simulink model "aerobalancin_modelo"  (R2025b)
settings: Solver=VariableStepAuto  StartTime=0.0  StopTime=40  FixedStep=1e-5  RelTol=1e-3
values from neighbouring files (symbols this model uses):
  d1 = 130.5e-3    (= 0.1305)    [Fuerzas.m]    (also in hinf.m)
  I = 1.3636e-4    (= 0.00013636)    [Fuerzas.m]    (also in hinf.m)
  k = (Wcp*d2-d1*Wm-e*Wb)    (= -0.00869250366)    [Fuerzas.m]    (also in hinf.m)
  Ka = m    (= 0.00012984)    [hinf.m]
  Kb = b    (= -0.0231)    [hinf.m]
  mu = 2e-04    (= 0.0002)    [Fuerzas.m]    (also in hinf.m = 0.0004)
  P_pwm_deg = series(Scale * P0, Act)    [hinf.m]
  T_ref = feedback(K*P_pwm_deg, 1)    [hinf.m]
undefined symbols (not defined in the file or in its folder): K
libraries: simulink_extras x3
settings Model: Creator=Gabriel Bojaca  LastModifiedBy=Gabriel Bojaca

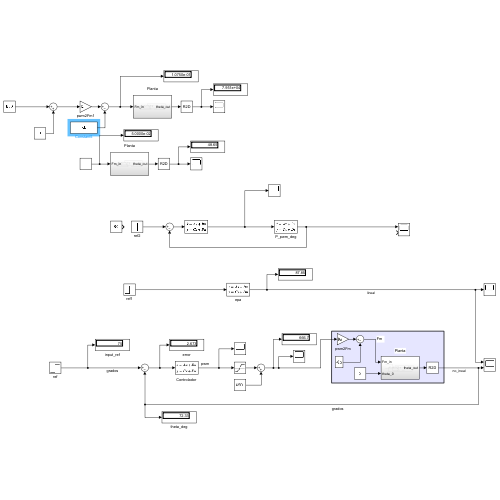
[thumbnail: Simulink's stored preview of the top-level diagram]
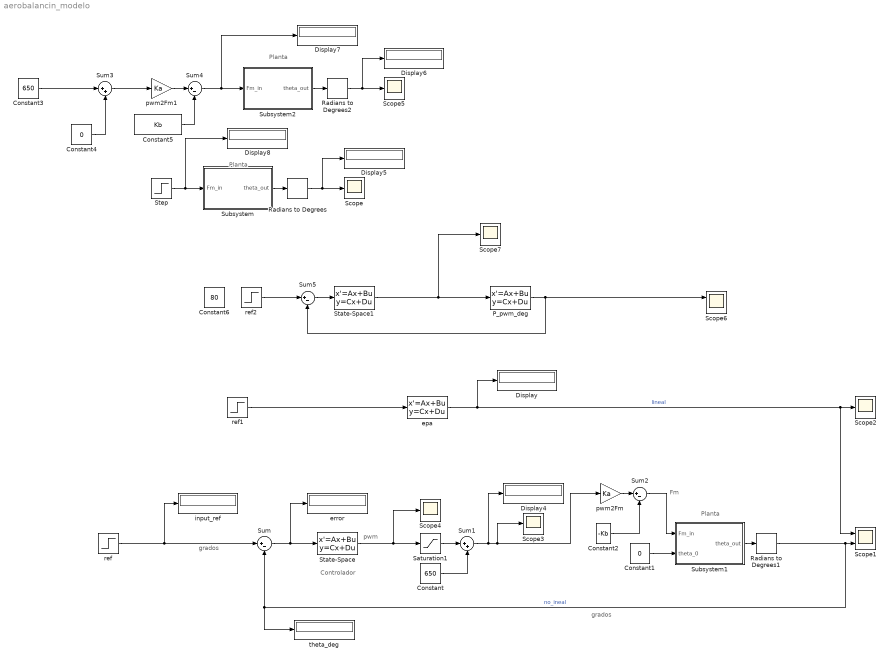
== system aerobalancin_modelo ==
  note: pwm
  note: Fm
  note: grados
  note: grados
  note: Planta
  note: Planta
  note: Controlador
  note: Planta
  Constant : Constant  Value=650
  Constant1 : Constant  Value=0
  Constant2 : Constant  Value=-Kb
  Constant3 : Constant  Value=650
  Constant4 : Constant  Value=0
  Constant5 : Constant  Value=Kb
  Constant6 : Constant  Value=80
  Display{,4..8} (6 alike) : Display
      Display7 settings: Format=short_e
      Display8 settings: Format=short_e
  P_pwm_deg : StateSpace  A=P_pwm_deg.A  B=P_pwm_deg.B  C=P_pwm_deg.C  D=P_pwm_deg.D  InitialCondition=0
  Radians to Degrees : simulink_extras/Transformations/Radians to Degrees
  Radians to Degrees1 : simulink_extras/Transformations/Radians to Degrees
  Radians to Degrees2 : simulink_extras/Transformations/Radians to Degrees
  Saturation1 : Saturate  UpperLimit=1023  LowerLimit=-1023  ZeroCross=off
  Scope{,2..5,7} (6 alike) : Scope
      Scope settings: ActiveDisplayYMinimum=-1  ActiveDisplayYMaximum=1
      Scope2 settings: ActiveDisplayYMinimum=79.481508887429072  ActiveDisplayYMaximum=97.233534907130334  DataLoggingVariableName=ScopeData2
      Scope3 settings: ActiveDisplayYMinimum=-1  ActiveDisplayYMaximum=1  DataLoggingVariableName=ScopeData3
      Scope4 settings: ActiveDisplayYMinimum=-86.058155781433356  ActiveDisplayYMaximum=157.82486783945171  DataLoggingVariableName=ScopeData4
      Scope5 settings: ActiveDisplayYMinimum=-227.29137035999565  ActiveDisplayYMaximum=925.661296141076  DataLoggingVariableName=ScopeData5
      Scope7 settings: ActiveDisplayYMinimum=-379.74870159092234  ActiveDisplayYMaximum=1124.590386355748  DataLoggingVariableName=ScopeData7
  Scope1 : Scope  NumInputPorts=2
      settings: ActiveDisplayYMinimum=-12.36574518282506  ActiveDisplayYMaximum=111.29170664542558
  Scope6 : Scope  NumInputPorts=2
      settings: ActiveDisplayYMinimum=-21.487013415649258  ActiveDisplayYMaximum=193.38312074084337  DataLoggingVariableName=ScopeData6
  State-Space : StateSpace  A=K.A  B=K.B  C=K.C  D=K.D  InitialCondition=0
  State-Space1 : StateSpace  A=K.A  B=K.B  C=K.C  D=K.D  InitialCondition=0
  Step : Step  After=50e-3  SampleTime=0
  Subsystem : Subsystem
  Subsystem1 : Subsystem
  Subsystem2 : Subsystem
  Sum{,2,4..5} (4 alike) : Sum  Inputs=|+-
  Sum1 : Sum  Inputs=|++
  Sum3 : Sum  Inputs=|++
  epa : StateSpace  A=T_ref.A  B=T_ref.B  C=T_ref.C  D=T_ref.D  InitialCondition=0
  error : Display
  input_ref : Display
  pwm2Fm : Gain  Gain=Ka
  pwm2Fm1 : Gain  Gain=Ka
  ref : Step  Time=20  Before=60  After=75  SampleTime=0
  ref1 : Step  Time=10  Before=77  After=85  SampleTime=0
  ref2 : Step  Time=0  Before=77  After=85  SampleTime=0
  theta_deg : Display
  wires:
  Subsystem/1(theta_out) -> Radians to Degrees/1
  Step/1 -> Display8/1, Subsystem/1(Fm_in)
  Subsystem1/1(theta_out) -> Radians to Degrees1/1
  Sum/1 -> State-Space/1, error/1
  Radians to Degrees1/1 -> Sum/2, theta_deg/1, Scope1/2  "no_ineal"
  ref/1 -> Sum/1, input_ref/1
  epa/1 -> Display/1, Scope1/1, Scope2/1  "lineal"
  State-Space/1 -> Saturation1/1, Scope4/1
  Sum1/1 -> Display4/1, pwm2Fm/1, Scope3/1
  Constant/1 -> Sum1/2
  Constant1/1 -> Subsystem1/2(theta_0)
  pwm2Fm/1 -> Sum2/1
  Sum2/1 -> Subsystem1/1(Fm_in)
  Constant2/1 -> Sum2/2
  Radians to Degrees/1 -> Display5/1, Scope/1
  Subsystem2/1(theta_out) -> Radians to Degrees2/1
  Radians to Degrees2/1 -> Display6/1, Scope5/1
  Sum4/1 -> Display7/1, Subsystem2/1(Fm_in)
  Sum3/1 -> pwm2Fm1/1
  Constant3/1 -> Sum3/1
  Constant4/1 -> Sum3/2
  pwm2Fm1/1 -> Sum4/1
  Constant5/1 -> Sum4/2
  ref1/1 -> epa/1
  Sum5/1 -> State-Space1/1
  P_pwm_deg/1 -> Sum5/2, Scope6/1
  ref2/1 -> Sum5/1
  Saturation1/1 -> Sum1/1
  State-Space1/1 -> P_pwm_deg/1, Scope7/1

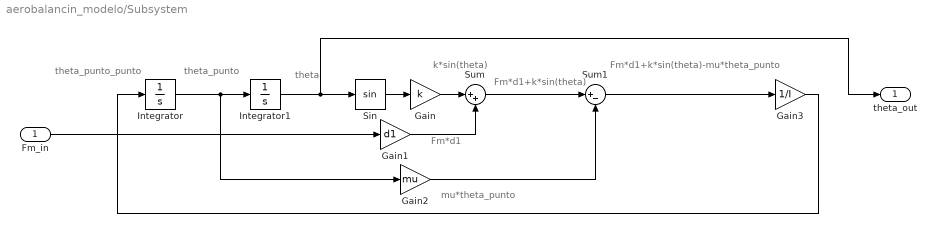
== system aerobalancin_modelo/Subsystem ==
  note: Fm*d1
  note: k*sin(theta)
  note: theta_punto_punto
  note: theta_punto
  note: theta
  note: Fm*d1+k*sin(theta)
  note: mu*theta_punto
  note: Fm*d1+k*sin(theta)-mu*theta_punto
  Fm_in : Inport
  Gain : Gain  Gain=k
  Gain1 : Gain  Gain=d1
  Gain2 : Gain  Gain=mu
  Gain3 : Gain  Gain=1/I
  Integrator : Integrator
  Integrator1 : Integrator
  Sin : Trigonometry
  Sum : Sum  Inputs=|++
  Sum1 : Sum  Inputs=|+-
  theta_out : Outport
  wires:
  Sum1/1 -> Gain3/1
  Gain3/1 -> Integrator/1
  Sin/1 -> Gain/1
  Integrator/1 -> Gain2/1, Integrator1/1
  Integrator1/1 -> theta_out/1, Sin/1
  Gain/1 -> Sum/1
  Sum/1 -> Sum1/1
  Gain2/1 -> Sum1/2
  Gain1/1 -> Sum/2
  Fm_in/1 -> Gain1/1

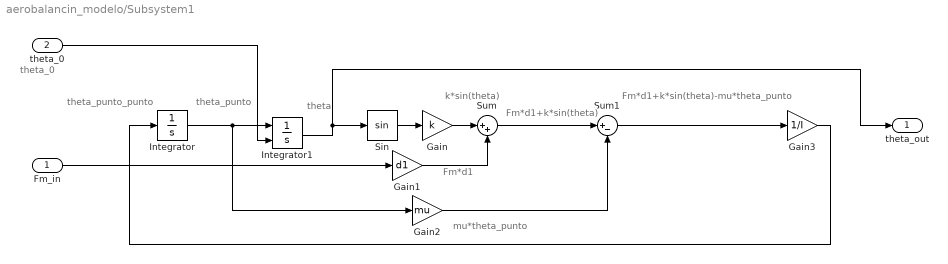
== system aerobalancin_modelo/Subsystem1 ==
  note: theta_0
  note: Fm*d1
  note: k*sin(theta)
  note: theta_punto_punto
  note: theta_punto
  note: theta
  note: Fm*d1+k*sin(theta)
  note: mu*theta_punto
  note: Fm*d1+k*sin(theta)-mu*theta_punto
  Fm_in : Inport
  theta_0 : Inport  Port=2
  Gain : Gain  Gain=k
  Gain1 : Gain  Gain=d1
  Gain2 : Gain  Gain=mu
  Gain3 : Gain  Gain=1/I
  Integrator : Integrator
  Integrator1 : Integrator  InitialConditionSource=external  InitialCondition=deg2rad(80)*0
  Sin : Trigonometry
  Sum : Sum  Inputs=|++
  Sum1 : Sum  Inputs=|+-
  theta_out : Outport
  wires:
  Sum1/1 -> Gain3/1
  Gain3/1 -> Integrator/1
  Sin/1 -> Gain/1
  Integrator/1 -> Gain2/1, Integrator1/1
  Integrator1/1 -> theta_out/1, Sin/1
  Gain/1 -> Sum/1
  Sum/1 -> Sum1/1
  Gain2/1 -> Sum1/2
  Gain1/1 -> Sum/2
  Fm_in/1 -> Gain1/1
  theta_0/1 -> Integrator1/2

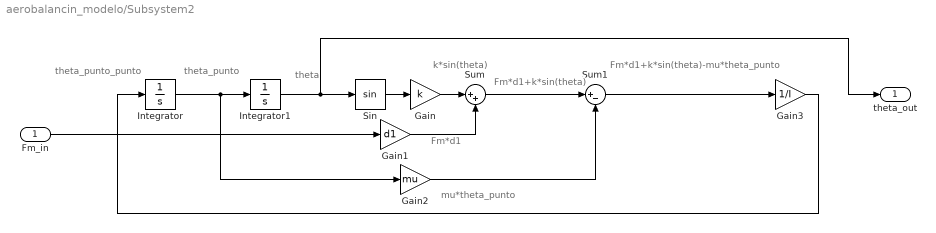
== system aerobalancin_modelo/Subsystem2 ==
  note: Fm*d1
  note: k*sin(theta)
  note: theta_punto_punto
  note: theta_punto
  note: theta
  note: Fm*d1+k*sin(theta)
  note: mu*theta_punto
  note: Fm*d1+k*sin(theta)-mu*theta_punto
  Fm_in : Inport
  Gain : Gain  Gain=k
  Gain1 : Gain  Gain=d1
  Gain2 : Gain  Gain=mu
  Gain3 : Gain  Gain=1/I
  Integrator : Integrator
  Integrator1 : Integrator
  Sin : Trigonometry
  Sum : Sum  Inputs=|++
  Sum1 : Sum  Inputs=|+-
  theta_out : Outport
  wires:
  Sum1/1 -> Gain3/1
  Gain3/1 -> Integrator/1
  Sin/1 -> Gain/1
  Integrator/1 -> Gain2/1, Integrator1/1
  Integrator1/1 -> theta_out/1, Sin/1
  Gain/1 -> Sum/1
  Sum/1 -> Sum1/1
  Gain2/1 -> Sum1/2
  Gain1/1 -> Sum/2
  Fm_in/1 -> Gain1/1
